simulink model "Subsystem2"  (R2020b)
settings: Solver=VariableStepAuto  StartTime=0.0  StopTime=120  RelTol=1e-3
values from neighbouring files (symbols this model uses):
  b = 50.0    [CruiseDict.sldd]
  m = 1000.0    [CruiseDict.sldd]
settings Model: DataDictionary=CruiseDict.sldd  Creator=DELL  LastModifiedBy=DELL
settings DataIOCC: SaveOutput=off  SaveTime=off

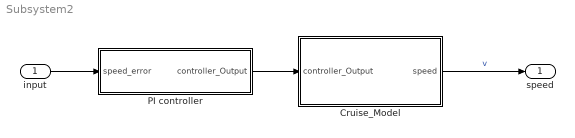
== system Subsystem2 ==
  input : Inport  OutDataTypeStr=double  PortDimensions=1  SampleTime=0
  Cruise_Model : Subsystem
  PI controller : Subsystem
  speed : Outport  OutDataTypeStr=double  PortDimensions=1  SampleTime=0
  wires:
  PI controller/1(controller_Output) -> Cruise_Model/1(controller_Output)
  Cruise_Model/1(speed) -> speed/1  "v"
  input/1 -> PI controller/1(speed_error)

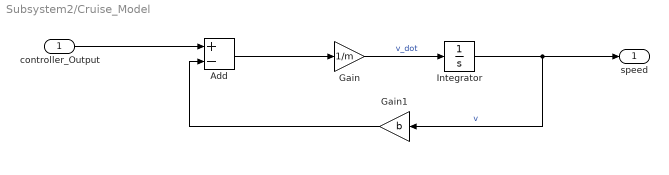
== system Subsystem2/Cruise_Model ==
  controller_Output : Inport
  Add : Sum  Inputs=+-
  Gain : Gain  Gain=1/m
  Gain1 : Gain  Gain=b
  Integrator : Integrator
  speed : Outport
  wires:
  controller_Output/1 -> Add/1
  Integrator/1 -> Gain1/1, speed/1  "v"
  Gain/1 -> Integrator/1  "v_dot"
  Gain1/1 -> Add/2
  Add/1 -> Gain/1

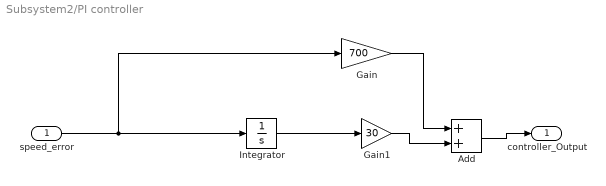
== system Subsystem2/PI controller ==
  speed_error : Inport
  Add : Sum
  Gain : Gain  Gain=700
  Gain1 : Gain  Gain=30
  Integrator : Integrator
  controller_Output : Outport
  wires:
  speed_error/1 -> Integrator/1, Gain/1
  Integrator/1 -> Gain1/1
  Gain/1 -> Add/1
  Add/1 -> controller_Output/1
  Gain1/1 -> Add/2
